simulink model "SamplingAndReconstruction"  (R2023a)
settings: Solver=VariableStepAuto  StartTime=0.0  StopTime=5  RelTol=1e-3
libraries: dspfdesign x1, dspsigops x1
settings Model: Creator=Admin  LastModifiedBy=Admin

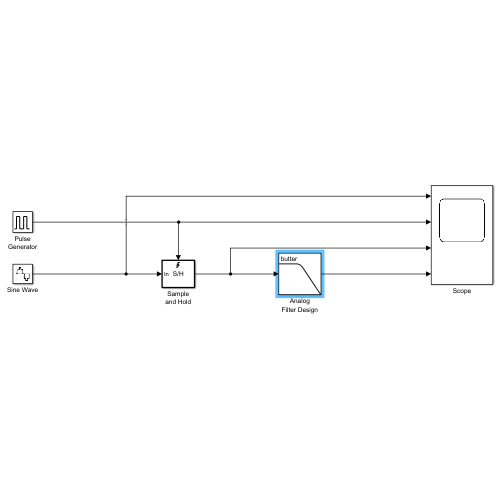
[thumbnail: Simulink's stored preview of the top-level diagram]
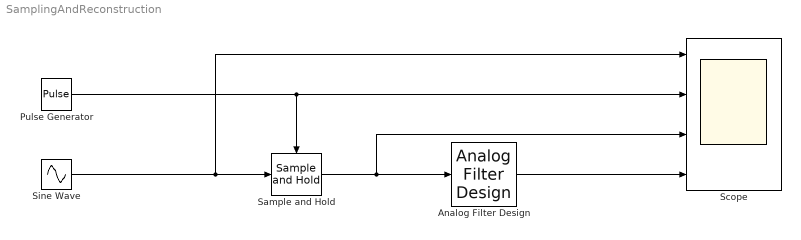
== system SamplingAndReconstruction ==
  Analog Filter Design : dspfdesign/Analog Filter Design  method=Butterworth  filttype=Lowpass  N=4  Wlo=2*pi*10  Whi=80  Rp=2  Rs=40
  Pulse Generator : DiscretePulseGenerator  PulseType=Time based  Amplitude=5  Period=0.001  PulseWidth=50
  Sample and Hold : dspsigops/Sample and Hold  trig=Rising edge  initCond=0  latchinput=off
  Scope : Scope  NumInputPorts=4
  Sine Wave : Sin  Amplitude=5  Frequency=2*pi*10  SampleTime=1/100000
  wires:
  Sine Wave/1 -> Scope/1, Sample and Hold/1
  Pulse Generator/1 -> Scope/2, Sample and Hold/Trigger
  Sample and Hold/1 -> Scope/3, Analog Filter Design/1
  Analog Filter Design/1 -> Scope/4
